simulink library "SLUGS_Library"  (Simulink 7.8)
settings: Solver=ode45  SolverMode=SingleTasking  StartTime=0.0  StopTime=10.0  RelTol=1e-3
values from neighbouring files (symbols this model uses):
  apSampleTime = 0.01    [mcuInit.m]
  derivativesConstant = 5    [mcuInit.m]
  latlong_WP = 1    [mcuInit.m]
  T = 0.01    [mcuInit.m]
  Xpoints = [0 0]    [mcuInit.m]
  Ypoints = [0 0]    [mcuInit.m]
  Zpoints = [0 0]    [mcuInit.m]
undefined symbols (not defined in the file or in its folder): bankCommandLimit, barAdjust, baroCutTemp, baroOffset, baroScale, barTGain1, barTGain2, barTMean1, barTMean2, baseHeight, baseTemp, daLimit, deLimit, DiscIntNeverNeededParam, drLimit, dtLimit, gaind, getGSLocation, getWP, GS_location, Init_onlyOnce, Init_Reset, IPStar, ISA_g, lapseRate, mass, maxAcc, MaxDwnPthStar, maxDynPressure, maxEta, Ndelay, param, pitAdjust, pitchCommandLimit, pitCutTemp, pitotOffset, pitotScale, pitTGain1, pitTGain2, pitTMean1, pitTMean2, polesd, pressureSensorCutoff, rollControlLimit, SampleT, setDiagnosticFloat, setDiagnosticShort, setLogFloat1, setLogFloat2, setNavLong, setNavNav, tanIntercept, Ts, u1, y1, yawDamperLimit, yo, zerosd
libraries: SLUGS_Library x90, simulink x37, dsPICdrivers x33, aerolibconvert2 x4, aerolibutil x1, aerolibobsolete x1
(part 2 of 7)

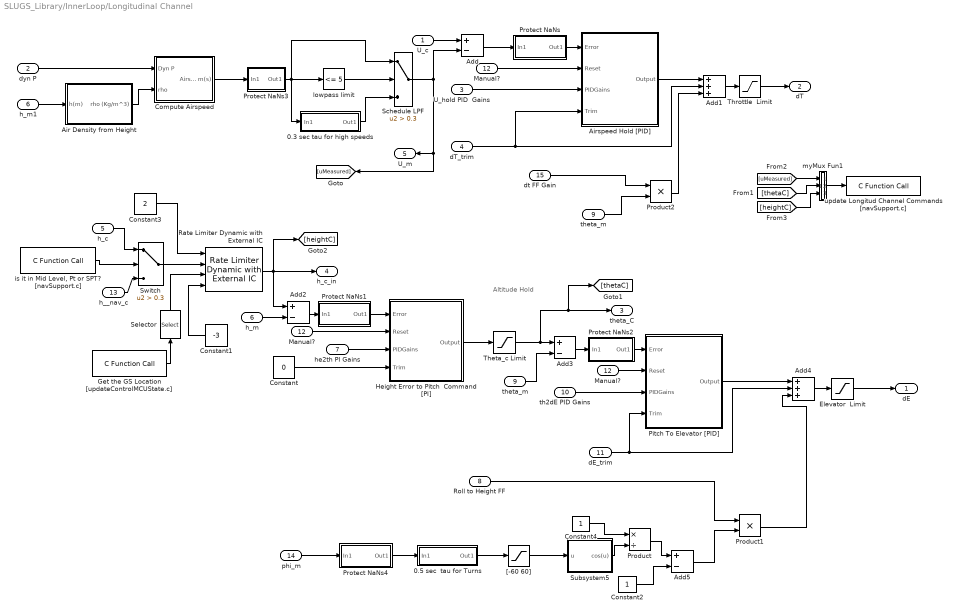
== system SLUGS_Library/InnerLoop/Longitudinal Channel ==
  note: Altitude Hold
  U_c : Inport
  dyn P : Inport  Port=2
  U_hold PID  Gains : Inport  Port=3
  dT_trim : Inport  Port=4
  h_c : Inport  Port=5
  h_m : Inport  Port=6
  he2th PI Gains : Inport  Port=7
  Roll to Height FF : Inport  Port=8
  theta_m : Inport  Port=9
  th2dE PID Gains : Inport  Port=10
  dE_trim : Inport  Port=11
  Manual? : Inport  Port=12
  h__nav_c : Inport  Port=13
  phi_m : Inport  Port=14
  dt FF Gain : Inport  Port=15
  " 0.3 sec tau for high speeds" : Subsystem  mask(Tustin1stOrderLowpassAutoInitialCondition){f=1, T=T}
      mask prompts: f "Lowpass Frequency"; T "Sample Time"
      mask help: Takes a 3db rolloff frequency (in Hz, NOT radians/s) and a sample time. Performs a symbolic Tustin conversion and implements in a discrete filter. The initial output of the filter is set by the first sample.
      mask Help: Enter the desired 3db rolloff frequency in Hz and the sample time. Initial conditions are sampled automatically.
      mask Display: fprintf('%.2f Hz lowpass',f)
  0.5 sec  tau for Turns : Subsystem  mask(Tustin1stOrderLowpassAutoInitialCondition){f=0.32, T=T}
      mask prompts: f "Lowpass Frequency"; T "Sample Time"
      mask help: Takes a 3db rolloff frequency (in Hz, NOT radians/s) and a sample time. Performs a symbolic Tustin conversion and implements in a discrete filter. The initial output of the filter is set by the first sample.
      mask Help: Enter the desired 3db rolloff frequency in Hz and the sample time. Initial conditions are sampled automatically.
      mask Display: fprintf('%.2f Hz lowpass',f)
  Add : Sum  Inputs=+-
  Add1 : Sum  Inputs=3  OutDataTypeStr=single
  Add2 : Sum  Inputs=+-  OutDataTypeStr=single
  Add3 : Sum  Inputs=+-  OutDataTypeStr=single
  Add4 : Sum  Inputs=3  OutDataTypeStr=single
  Add5 : Sum  Inputs=+-  OutDataTypeStr=single
  Air Density from Height : Subsystem  AncestorBlock=SLUGS_Library/Air Density from Height
  Airspeed Hold [PID] : Subsystem  AncestorBlock=SLUGS_Library/Control Blocks/PID Controller w//Anti-Windup  mask(PID){Tsample=apSampleTime, Ndelay=derivativesConstant, upperSaturationLimit=dtLimit, lowerSaturationLimit=0}
      mask prompts: Tsample "Sample Time"; Ndelay "Integer delays for de/dt"; upperSaturationLimit "Upper Saturation Limit"; lowerSaturationLimit "Lower Saturation Limit"
      mask help: PID controller block with anti-windup and saturation limits. Implemented as a discrete forwardl integration which stops integrating when the output is saturated. Derivative is implemented as a numerical derivative with N integer delays to smooth output.
      mask Display:
      | disp('PID')
      | port_label('input',1,'error')
      | port_label('input',3,'gains')
      | port_label('input',2,'reset')
      | port_label('input',4,'trim')
      | port_label('output',1,'output')
  Compute Airspeed : Subsystem  AncestorBlock=SLUGS_Library/Compute Airspeed
  Constant : Constant  Value=0
  Constant1 : Constant  Value=-3  OutDataTypeStr=single
  Constant2 : Constant  OutDataTypeStr=single
  Constant3 : Constant  Value=2  OutDataTypeStr=single
  Constant4 : Constant  OutDataTypeStr=single
  Elevator  Limit : Saturate  UpperLimit=deLimit  LowerLimit=-deLimit  SampleTime=apSampleTime
  Get the GS Location [updateControlMCUState.c] : dsPICdrivers/OTHERS/C Function Call  Tag=dsPIC_dsPIC_CFunctionCall  FctUpdate=Output Function  fctName='getGSLocation'  INPUT_SIZE=1  INPUT1=--  INPUT2=--  INPUT3=--  OUTPUT_SIZE=3  OUTPUT1=real32  SampleTime=0.01  InputType=[ ]  OutputType=[ 7 ]  FctDeclaration=extern void getGSLocation(real32_T* y1);  FctCall=getGSLocation(*%y1);  OrderingInOutPopup=None  FctStart=None  FctStart_Name=Init_onlyOnce  FctStart_Declaration=inline extern void Init_onlyOnce();  FctStart_Call=Init_onlyOnce();  FctInit=None  FctInit_Name=Init_Reset  FctInit_Declaration=inline extern void Init_Reset();  FctInit_Call=Init_Reset();  PinDigitalInput=[]  PinDigitalOutput=[]  AnalogueInput=[]
  Height Error to Pitch  Command [PI] : Subsystem  AncestorBlock=SLUGS_Library/Control Blocks/PI Controller w//Anti-Windup  mask(PID){Tsample=apSampleTime, Ndelay=derivativesConstant, upperSaturationLimit=pitchCommandLimit, lowerSaturationLimit=-pitchCommandLimit}
      mask prompts: Tsample "Sample Time"; Ndelay "Integer delays for de/dt"; upperSaturationLimit "Upper Saturation Limit"; lowerSaturationLimit "Lower Saturation Limit"
      mask help: PID controller block with anti-windup and saturation limits. Implemented as a discrete forwardl integration which stops integrating when the output is saturated. Derivative is implemented as a numerical derivative with N integer delays to smooth output.
      mask Display:
      | disp('PI')
      | port_label('input',1,'error')
      | port_label('input',3,'gains')
      | port_label('input',2,'reset')
      | port_label('input',4,'trim')
      | port_label('output',1,'output')
  "Manual? " : InportShadow  Port=12
  "Manual?  " : InportShadow  Port=12
  Pitch To Elevator [PID] : Subsystem  AncestorBlock=SLUGS_Library/Control Blocks/PID Controller w//Anti-Windup  mask(PID){Tsample=apSampleTime, Ndelay=derivativesConstant, upperSaturationLimit=deLimit, lowerSaturationLimit=-deLimit}
      mask prompts: Tsample "Sample Time"; Ndelay "Integer delays for de/dt"; upperSaturationLimit "Upper Saturation Limit"; lowerSaturationLimit "Lower Saturation Limit"
      mask help: PID controller block with anti-windup and saturation limits. Implemented as a discrete forwardl integration which stops integrating when the output is saturated. Derivative is implemented as a numerical derivative with N integer delays to smooth output.
      mask Display:
      | disp('PID')
      | port_label('input',1,'error')
      | port_label('input',3,'gains')
      | port_label('input',2,'reset')
      | port_label('input',4,'trim')
      | port_label('output',1,'output')
  Product : Product  Inputs=*/  RndMeth=Zero
  Product1 : Product  RndMeth=Zero
  Product2 : Product  RndMeth=Zero
  Protect NaNs : Subsystem
  Protect NaNs1 : Subsystem
  Protect NaNs2 : Subsystem
  Protect NaNs3 : Subsystem
  Protect NaNs4 : Subsystem
  Rate Limiter Dynamic with External IC : SLUGS_Library/Singnal Routing & Conditioning/Rate Limiter Dynamic with External IC  rlIC=0
  Schedule LPF : Switch  Criteria=u2 > Threshold  Threshold=0.3
  Selector : Selector  InputPortWidth=3  IndexOptions=Index vector (dialog)  Indices=[1 ]  OutputSizes=1
  Subsystem5 : Subsystem  AncestorBlock=SLUGS_Library/Subsystem5
  Switch : Switch  Criteria=u2 > Threshold  Threshold=0.3  OutDataTypeStr=Inherit: Inherit via back propagation  InputSameDT=on
  Theta_c Limit : Saturate  UpperLimit=pitchCommandLimit  LowerLimit=-pitchCommandLimit  SampleTime=apSampleTime
  Throttle  Limit : Saturate  UpperLimit=dtLimit  LowerLimit=0  SampleTime=apSampleTime
  "[-60 60]" : Saturate  UpperLimit=60  LowerLimit=-60  SampleTime=apSampleTime
  h_m1 : InportShadow  Port=6
  "is it in Mid Level, Pt or SPT? [navSupport.c]" : dsPICdrivers/OTHERS/C Function Call  Tag=dsPIC_dsPIC_CFunctionCall  FctUpdate=Output Function  fctName='isPassthrough'  INPUT_SIZE=1  INPUT1=--  INPUT2=--  INPUT3=--  OUTPUT_SIZE=1  OUTPUT1=uint8  SampleTime=0.01  InputType=[ ]  OutputType=[ 2 ]  FctDeclaration=extern uint8_T isPassthrough();  FctCall=%y1 = isPassthrough();  OrderingInOutPopup=None  FctStart=None  FctStart_Name=Init_onlyOnce  FctStart_Declaration=inline extern void Init_onlyOnce();  FctStart_Call=Init_onlyOnce();  FctInit=None  FctInit_Name=Init_Reset  FctInit_Declaration=inline extern void Init_Reset();  FctInit_Call=Init_Reset();  PinDigitalInput=[]  PinDigitalOutput=[]  AnalogueInput=[]
  lowpass limit : simulink/Logic and Bit Operations/Compare To Constant  relop=<=  const=5  OutDataTypeStr=uint8  ZeroCross=off
  myMux Fun1 : MATLAB Function  TreatAsAtomicUnit=on
  "theta_m " : InportShadow  Port=9
  update Longitud Channel Commands [navSupport.c] : dsPICdrivers/OTHERS/C Function Call  Tag=dsPIC_dsPIC_CFunctionCall  FctUpdate=Output Function  fctName='setNavLong'  INPUT_SIZE=3  INPUT1=real32  INPUT2=--  INPUT3=--  OUTPUT_SIZE=1  OUTPUT1=--  SampleTime=.01  InputType=[ 7 ]  OutputType=[ ]  FctDeclaration=extern void setNavLong(real32_T* u1);  FctCall=setNavLong(*%u1);  OrderingInOutPopup=None  FctStart=None  FctStart_Name=Init_onlyOnce  FctStart_Declaration=inline extern void Init_onlyOnce();  FctStart_Call=Init_onlyOnce();  FctInit=None  FctInit_Name=Init_Reset  FctInit_Declaration=inline extern void Init_Reset();  FctInit_Call=Init_Reset();  PinDigitalInput=[]  PinDigitalOutput=[]  AnalogueInput=[]
  dE : Outport
  dT : Outport  Port=2
  theta_C : Outport  Port=3
  h_c_in : Outport  Port=4
  U_m : Outport  Port=5
  wires:
  [heightC] -> myMux Fun1/3(u3)
  h_c/1 -> Switch/1
  h__nav_c/1 -> Switch/3
  Get the GS Location [updateControlMCUState.c]/1 -> Selector/1
  Protect NaNs4/1(Out1) -> 0.5 sec  tau for Turns/1(In1)
  Protect NaNs3/1(Out1) -> Schedule LPF/1, lowpass limit/1, " 0.3 sec tau for high speeds"/1(In1)
  Protect NaNs2/1(Out1) -> Pitch To Elevator [PID]/1(Error)
  Protect NaNs1/1(Out1) -> Height Error to Pitch  Command [PI]/1(Error)
  Protect NaNs/1(Out1) -> Airspeed Hold [PID]/1(Error)
  Constant/1 -> Height Error to Pitch  Command [PI]/4(Trim)
  U_hold PID  Gains/1 -> Airspeed Hold [PID]/3(PIDGains)
  dt FF Gain/1 -> Product2/1
  Product2/1 -> Add1/3
  "theta_m "/1 -> Product2/2
  Product1/1 -> Add4/3
  Roll to Height FF/1 -> Product1/1
  Add5/1 -> Product1/2
  "[-60 60]"/1 -> Subsystem5/1(u)
  0.5 sec  tau for Turns/1(Out1) -> "[-60 60]"/1
  Product/1 -> Add5/1
  Constant4/1 -> Product/1
  Subsystem5/1(cos(u)) -> Product/2
  Constant2/1 -> Add5/2
  phi_m/1 -> Protect NaNs4/1(In1)
  " 0.3 sec tau for high speeds"/1(Out1) -> Schedule LPF/3
  lowpass limit/1 -> Schedule LPF/2
  Compute Airspeed/1(Airspeed m(s)) -> Protect NaNs3/1(In1)
  Schedule LPF/1 -> [uMeasured], U_m/1, Add/2
  [thetaC] -> myMux Fun1/2(u2)
  [uMeasured] -> myMux Fun1/1(u1)
  myMux Fun1/1(y) -> update Longitud Channel Commands [navSupport.c]/1
  U_c/1 -> Add/1
  Add/1 -> Protect NaNs/1(In1)
  Airspeed Hold [PID]/1(Output) -> Add1/1
  dT_trim/1 -> Airspeed Hold [PID]/4(Trim), Add1/2
  Add1/1 -> Throttle  Limit/1
  Throttle  Limit/1 -> dT/1
  Add2/1 -> Protect NaNs1/1(In1)
  h_m/1 -> Add2/2
  theta_m/1 -> Add3/2
  Manual?/1 -> Airspeed Hold [PID]/2(Reset)
  "Manual? "/1 -> Height Error to Pitch  Command [PI]/2(Reset)
  "Manual?  "/1 -> Pitch To Elevator [PID]/2(Reset)
  Add4/1 -> Elevator  Limit/1
  Pitch To Elevator [PID]/1(Output) -> Add4/1
  dE_trim/1 -> Pitch To Elevator [PID]/4(Trim), Add4/2
  Elevator  Limit/1 -> dE/1
  Air Density from Height/1(rho (Kg/m^3)) -> Compute Airspeed/2(rho)
  dyn P/1 -> Compute Airspeed/1(Dyn P)
  h_m1/1 -> Air Density from Height/1(h(m))
  he2th PI Gains/1 -> Height Error to Pitch  Command [PI]/3(PIDGains)
  th2dE PID Gains/1 -> Pitch To Elevator [PID]/3(PIDGains)
  Add3/1 -> Protect NaNs2/1(In1)
  Theta_c Limit/1 -> [thetaC], theta_C/1, Add3/1
  "is it in Mid Level, Pt or SPT? [navSupport.c]"/1 -> Switch/2
  Rate Limiter Dynamic with External IC/1 -> [heightC], h_c_in/1, Add2/1
  Height Error to Pitch  Command [PI]/1(Output) -> Theta_c Limit/1
  Constant3/1 -> Rate Limiter Dynamic with External IC/1
  Switch/1 -> Rate Limiter Dynamic with External IC/2
  Selector/1 -> Rate Limiter Dynamic with External IC/3
  Constant1/1 -> Rate Limiter Dynamic with External IC/4

== system SLUGS_Library/InnerLoop/Navigation ==
  Puav : Inport  SampleTime=apSampleTime
  Max WP Idx : Inport  Port=2
  Vxyz : Inport  Port=3
  Start WP Idx : Inport  Port=4
  L1 Base (m) : Inport  Port=5
  R : Inport  Port=6
  WP Fly : Inport  Port=7
  Compute Lateral Error : SLUGS_Library/Navigation/Compute Lateral Error
  Compute WP Index : Subsystem  AncestorBlock=SLUGS_Library/Navigation/Compute WP Index
  Get Wps Compute Frenet : Subsystem
  "Park, Deyst & How Lat Accel Cmd" : SLUGS_Library/Navigation/Park, Deyst & How Lat Accel Cmd
  Selector : Selector  InputPortWidth=3  IndexOptions=Index vector (dialog)  Indices=[3]  OutputSizes=1
  To Workspace1 : ToWorkspace  VariableName=as_c  SampleTime=-1  SaveFormat=Array
  To Workspace2 : ToWorkspace  VariableName=N  SampleTime=-1  SaveFormat=Array
  To Workspace3 : ToWorkspace  VariableName=Phic  SampleTime=-1  SaveFormat=Array
  To Workspace4 : ToWorkspace  VariableName=T  SampleTime=-1  SaveFormat=Array
  UAV Weight : Constant  Value=mass  OutDataTypeStr=single
  UAV Pos1 : InportShadow  Port=1  SampleTime=apSampleTime
  as_c to phi_c : SLUGS_Library/Navigation/as_c to phi_c
  phi_c : Outport
  h_c : Outport  Port=2
  wires:
  Compute WP Index/2(WP0) -> Get Wps Compute Frenet/1(WP Idx 0)
  Compute WP Index/3(WP1) -> Get Wps Compute Frenet/2(WP Idx 1)
  Get Wps Compute Frenet/2(N) -> Compute Lateral Error/1, "Park, Deyst & How Lat Accel Cmd"/3, To Workspace2/1
  Get Wps Compute Frenet/1(T) -> To Workspace4/1, Compute WP Index/1(T1), "Park, Deyst & How Lat Accel Cmd"/2
  Puav/1 -> Compute WP Index/2(Puav)
  Max WP Idx/1 -> Compute WP Index/3(Max WP Index)
  Start WP Idx/1 -> Compute WP Index/4(StartingWP)
  "Park, Deyst & How Lat Accel Cmd"/1 -> To Workspace1/1, as_c to phi_c/1
  UAV Pos1/1 -> Compute Lateral Error/3
  as_c to phi_c/1 -> phi_c/1, To Workspace3/1
  UAV Weight/1 -> as_c to phi_c/2
  Compute Lateral Error/1 -> "Park, Deyst & How Lat Accel Cmd"/4
  Get Wps Compute Frenet/3(WP 1) -> Compute Lateral Error/2, Selector/1, Compute WP Index/5("WP1 ")
  Selector/1 -> h_c/1
  L1 Base (m)/1 -> "Park, Deyst & How Lat Accel Cmd"/5
  Compute WP Index/1(WP Change) -> Get Wps Compute Frenet/Enable
  R/1 -> Compute WP Index/6(R)
  Vxyz/1 -> "Park, Deyst & How Lat Accel Cmd"/1
  WP Fly/1 -> Compute WP Index/7(WP Fly)
  Compute WP Index/4(UAV IC) -> Get Wps Compute Frenet/3(UAV IC)

== system SLUGS_Library/Navigation/Bank to Psi Dot ==
  phi_c : Inport
  U_m : Inport  Port=2
  Constant1 : Constant  Value=9.80665  OutDataTypeStr=single
  Divide : Product  Inputs=/*  OutDataTypeStr=single
  Divide1 : Product  OutDataTypeStr=single
  Subsystem8 : SLUGS_Library/Subsystem8
  negprotect : MATLAB Function  TreatAsAtomicUnit=on
  psi_dot_c : Outport
  wires:
  U_m/1 -> negprotect/1(val)
  Constant1/1 -> Divide/2
  Divide1/1 -> psi_dot_c/1
  Subsystem8/1 -> Divide1/1
  phi_c/1 -> Subsystem8/1
  Divide/1 -> Divide1/2
  negprotect/1(zpVal) -> Divide/1

== system SLUGS_Library/Navigation/Compute Lateral Error ==
  N : Inport
  WP1 : Inport  Port=2
  UAV pos : Inport  Port=3
  Add : Sum  Inputs=+-
  Subsystem3 : SLUGS_Library/Subsystem3
  Pe_lat : Outport
  wires:
  WP1/1 -> Add/1
  UAV pos/1 -> Add/2
  N/1 -> Subsystem3/1
  Add/1 -> Subsystem3/2
  Subsystem3/1 -> Pe_lat/1

== system SLUGS_Library/Navigation/Compute Distance ==
  Pos 1 : Inport
  Pos 2 : Inport  Port=2
  Add : Sum  Inputs=+-
  Norm : SLUGS_Library/Navigation/Norm
  Dist : Outport
  wires:
  Pos 1/1 -> Add/1
  Pos 2/1 -> Add/2
  Add/1 -> Norm/1
  Norm/1 -> Dist/1

== system SLUGS_Library/Navigation/Compute Frenet ==
  Pos 1 : Inport
  Pos 2 : Inport  Port=2
  Add : Sum  Inputs=-+
  Normalize Vector : SLUGS_Library/Navigation/Normalize Vector
  "Normalize Vector " : SLUGS_Library/Navigation/Normalize Vector
  Select N  Terms : MATLAB Function  TreatAsAtomicUnit=on
  T : Outport
  N : Outport  Port=2
  wires:
  Pos 1/1 -> Add/1
  Pos 2/1 -> Add/2
  Add/1 -> Normalize Vector/1
  Normalize Vector/1 -> T/1, Select N  Terms/1(T)
  Select N  Terms/1(N) -> "Normalize Vector "/1
  "Normalize Vector "/1 -> N/1

== system SLUGS_Library/Navigation/Compute WP Index ==
  T1 : Inport
  Puav : Inport  Port=2
  Max WP Index : Inport  Port=3
  StartingWP : Inport  Port=4
  "WP1 " : Inport  Port=5
  R : Inport  Port=6
  WP Fly : Inport  Port=7
  Add : Sum  Inputs=2
  Compute Distance : SLUGS_Library/Navigation/Compute Distance
  Compute Modified L1 : Subsystem
  Data Type Conversion : DataTypeConversion  OutDataTypeStr=double  SampleTime=apSampleTime
  Embedded MATLAB Function : MATLAB Function  TreatAsAtomicUnit=on
  Enabled Subsystem : Subsystem  TreatAsAtomicUnit=on
  Hit  Crossing : HitCross  HitCrossingOffset=0.9  HitCrossingDirection=rising  SampleTime=apSampleTime
  IC : InitialCondition
  IC1 : InitialCondition  Value=0
  Integer Delay : Delay  DelayLength=1  InputProcessing=Inherited
  Integer Delay2 : Delay  DelayLength=1  InitialCondition=0  InputProcessing=Inherited
  Integer Delay3 : Delay  DelayLength=1  InitialCondition=150  InputProcessing=Inherited
  Logical Operator : Logic  Operator=OR  AllPortsSameDT=off  OutDataTypeStr=boolean
  "Puav " : InportShadow  Port=2
  Subsystem : Subsystem
  Switch Distance Less than? : RelationalOperator  OutDataTypeStr=boolean  SampleTime=apSampleTime
  WP1 1 : InportShadow  Port=5
  WP Change : Outport
  WP0 : Outport  Port=2
  WP1 : Outport  Port=3
  UAV IC : Outport  Port=4
  wires:
  Integer Delay/1 -> Compute Distance/2  "next WP"
  Puav/1 -> Compute Distance/1
  Embedded MATLAB Function/2(wp1) -> WP1/1
  Embedded MATLAB Function/1(wp0) -> WP0/1
  StartingWP/1 -> Embedded MATLAB Function/1(wpStart)
  Switch Distance Less than?/1 -> Data Type Conversion/1
  Max WP Index/1 -> Embedded MATLAB Function/2(wpCount)
  Compute Distance/1 -> Switch Distance Less than?/2
  "WP1 "/1 -> Integer Delay/1
  Hit  Crossing/1 -> Embedded MATLAB Function/3(swIncrement), IC/1
  Data Type Conversion/1 -> Hit  Crossing/1
  Embedded MATLAB Function/3(wp2) -> Compute Modified L1/3(WP2)
  WP1 1/1 -> Compute Modified L1/1(WP1)
  T1/1 -> Compute Modified L1/2(T1)
  Integer Delay2/1 -> Add/1
  Add/1 -> Compute Modified L1/Enable, Logical Operator/1
  IC/1 -> Add/2, Integer Delay2/1
  Compute Modified L1/1(P) -> Integer Delay3/1
  Integer Delay3/1 -> Switch Distance Less than?/1
  R/1 -> Compute Modified L1/4(R)
  WP Fly/1 -> IC1/1
  Subsystem/1(Just Enab) -> Enabled Subsystem/Enable, [WpEnabl]
  "Puav "/1 -> Enabled Subsystem/1(In1)
  Enabled Subsystem/1(Out1) -> UAV IC/1
  IC1/1 -> Subsystem/1(WP Fly)
  [WpEnabl] -> Embedded MATLAB Function/4(wpEnabl)
  Logical Operator/1 -> WP Change/1
  [WpEnabl] -> Logical Operator/2

== system SLUGS_Library/Navigation/Geod2LTP ==
  GS Lat,Lon : Inport
  GS ECEF : Inport  Port=2
  "Lat, deg(GPS)" : Inport  Port=3
  "Lon, deg(GPS)" : Inport  Port=4
  Hight,m(GPS) : Inport  Port=5
  ECEF2LTP (UEN) : Subsystem
      mask Display: plot(0,0,100,100,[45,40,35,40,40],[85,95,85,95,40],[85,95,85,95,40],[35,40,45,40,40],[60,40,10,20,10,14],[70,40,10,13,10,20],[56,45],[70,70],[60,60],[50,60],[60,60],[30,40],[50,60],[20,20],[30,40],[20,20],[45,55],[35,25],[75,65],[35,25])
  Geod2ECEF1 : Subsystem  mask{Re=6378137, Rp=6356752.3142}
      mask prompts: Re "Enter equatorial radius, m"; Rp "Enter polar radius,m"
  Mux : Mux  Inputs=3
  Reshape : Reshape  OutputDimensionality=Column vector (2-D)
  Reshape1 : Reshape
  Sum1 : Sum  Inputs=|+-  OutDataTypeStr=single  SaturateOnIntegerOverflow=on
  UEN 2 NEU : Gain  Gain=[0 0 1;0 1 0;1 0 0]  Multiplication=Matrix(K*u)  OutDataTypeStr=float('single')  SaturateOnIntegerOverflow=on  ParamDataTypeStr=Inherit: Same as input
  "NEU, m" : Outport
  wires:
  Reshape1/1 -> "NEU, m"/1
  Reshape/1 -> UEN 2 NEU/1
  Sum1/1 -> ECEF2LTP (UEN)/1(ECEF coordinates)
  Mux/1 -> Sum1/1  "r_mov"
  Hight,m(GPS)/1 -> Geod2ECEF1/1("height, m")
  ECEF2LTP (UEN)/1(Out) -> Reshape/1  "Moving Side"
  GS ECEF/1 -> Sum1/2
  GS Lat,Lon/1 -> ECEF2LTP (UEN)/2("Long, Lat")
  "Lon, deg(GPS)"/1 -> Geod2ECEF1/3(lon,deg)
  "Lat, deg(GPS)"/1 -> Geod2ECEF1/2("lat, deg")
  Geod2ECEF1/2("Ye, m ") -> Mux/2
  Geod2ECEF1/1("Xe, m ") -> Mux/1
  Geod2ECEF1/3("Ze, m ") -> Mux/3
  UEN 2 NEU/1 -> Reshape1/1

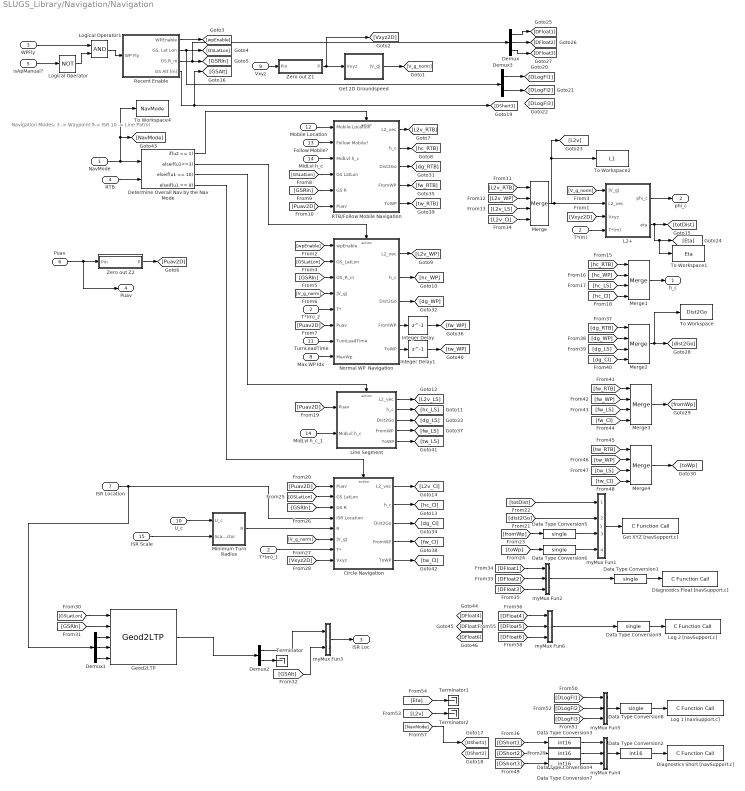
== system SLUGS_Library/Navigation/Navigation ==
  note: Navigation Modes:
      | 3 -> Waypoint
      | 9-> ISR
      | 10 -> Line Patrol
  NavMode : Inport
  T*(m) : Inport  Port=2
  WPFly : Inport  Port=3
  RTB : Inport  Port=4
  isApManual? : Inport  Port=5
  Puav : Inport  Port=6  SampleTime=apSampleTime
  ISR Location : Inport  Port=7
  Max WP Idx : Inport  Port=8
  Vxyz : Inport  Port=9  SampleTime=apSampleTime
  U_c : Inport  Port=10
  TurnLeadTime : Inport  Port=11
  Mobile Location : Inport  Port=12
  Follow Mobile? : Inport  Port=13
  MidLvl h_c : Inport  Port=14
  ISR Scale : Inport  Port=15
  Circle Navigation : Subsystem  TreatAsAtomicUnit=on
  Data Type Conversion{1,5..6,8..9} (5 alike) : DataTypeConversion  OutDataTypeStr=single
  Data Type Conversion{2..4,7} (4 alike) : DataTypeConversion  OutDataTypeStr=int16
  Demux : Demux  Outputs=3
  Demux1 : Demux  Outputs=3
  Demux2 : Demux  Outputs=[2 1]
  Demux3 : Demux  Outputs=2
  Determine Overall Nav by the Nav Mode : If  NumInputs=2  IfExpression=u2 == 1  ElseIfExpressions=u1==3, u1 == 10, u1 == 9  ShowElse=off
  Diagnostics Float [navSupport.c] : dsPICdrivers/OTHERS/C Function Call  Tag=dsPIC_dsPIC_CFunctionCall  FctUpdate=Output Function  fctName='setDiagnosticFloat'  INPUT_SIZE=3  INPUT1=real32  INPUT2=--  INPUT3=--  OUTPUT_SIZE=1  OUTPUT1=--  SampleTime=.01  InputType=[ 7 ]  OutputType=[ ]  FctDeclaration=extern void setDiagnosticFloat(real32_T* u1);  FctCall=setDiagnosticFloat(*%u1);  OrderingInOutPopup=None  FctStart=None  FctStart_Name=Init_onlyOnce  FctStart_Declaration=inline extern void Init_onlyOnce();  FctStart_Call=Init_onlyOnce();  FctInit=None  FctInit_Name=Init_Reset  FctInit_Declaration=inline extern void Init_Reset();  FctInit_Call=Init_Reset();  PinDigitalInput=[]  PinDigitalOutput=[]  AnalogueInput=[]
  Diagnostics Short [navSupport.c] : dsPICdrivers/OTHERS/C Function Call  Tag=dsPIC_dsPIC_CFunctionCall  FctUpdate=Output Function  fctName='setDiagnosticShort'  INPUT_SIZE=3  INPUT1=int16  INPUT2=--  INPUT3=--  OUTPUT_SIZE=1  OUTPUT1=--  SampleTime=.01  InputType=[ 3 ]  OutputType=[ ]  FctDeclaration=extern void setDiagnosticShort(int16_T* u1);  FctCall=setDiagnosticShort(*%u1);  OrderingInOutPopup=None  FctStart=None  FctStart_Name=Init_onlyOnce  FctStart_Declaration=inline extern void Init_onlyOnce();  FctStart_Call=Init_onlyOnce();  FctInit=None  FctInit_Name=Init_Reset  FctInit_Declaration=inline extern void Init_Reset();  FctInit_Call=Init_Reset();  PinDigitalInput=[]  PinDigitalOutput=[]  AnalogueInput=[]
  Geod2LTP : SLUGS_Library/Navigation/Geod2LTP
  Get 2D Groundspeed : Subsystem
  Get XYZ [navSupport.c] : dsPICdrivers/OTHERS/C Function Call  Tag=dsPIC_dsPIC_CFunctionCall  FctUpdate=Output Function  fctName='setNavNav'  INPUT_SIZE=4  INPUT1=real32  INPUT2=--  INPUT3=--  OUTPUT_SIZE=1  OUTPUT1=--  SampleTime=.01  InputType=[ 7 ]  OutputType=[ ]  FctDeclaration=extern void setNavNav(real32_T* u1);  FctCall=setNavNav(*%u1);  OrderingInOutPopup=None  FctStart=None  FctStart_Name=Init_onlyOnce  FctStart_Declaration=inline extern void Init_onlyOnce();  FctStart_Call=Init_onlyOnce();  FctInit=None  FctInit_Name=Init_Reset  FctInit_Declaration=inline extern void Init_Reset();  FctInit_Call=Init_Reset();  PinDigitalInput=[]  PinDigitalOutput=[]  AnalogueInput=[]
  Integer Delay : Delay  DelayLength=1  InputProcessing=Inherited
  Integer Delay1 : Delay  DelayLength=1  InputProcessing=Inherited
  L2+ : Subsystem
  Line Segment : Subsystem  TreatAsAtomicUnit=on
  Log 1 [navSupport.c] : dsPICdrivers/OTHERS/C Function Call  Tag=dsPIC_dsPIC_CFunctionCall  FctUpdate=Output Function  fctName='setLogFloat1'  INPUT_SIZE=3  INPUT1=real32  INPUT2=--  INPUT3=--  OUTPUT_SIZE=1  OUTPUT1=--  SampleTime=.01  InputType=[ 7 ]  OutputType=[ ]  FctDeclaration=extern void setLogFloat1(real32_T* u1);  FctCall=setLogFloat1(*%u1);  OrderingInOutPopup=None  FctStart=None  FctStart_Name=Init_onlyOnce  FctStart_Declaration=inline extern void Init_onlyOnce();  FctStart_Call=Init_onlyOnce();  FctInit=None  FctInit_Name=Init_Reset  FctInit_Declaration=inline extern void Init_Reset();  FctInit_Call=Init_Reset();  PinDigitalInput=[]  PinDigitalOutput=[]  AnalogueInput=[]
  Log 2 [navSupport.c] : dsPICdrivers/OTHERS/C Function Call  Tag=dsPIC_dsPIC_CFunctionCall  FctUpdate=Output Function  fctName='setLogFloat2'  INPUT_SIZE=3  INPUT1=real32  INPUT2=--  INPUT3=--  OUTPUT_SIZE=1  OUTPUT1=--  SampleTime=.01  InputType=[ 7 ]  OutputType=[ ]  FctDeclaration=extern void setLogFloat2(real32_T* u1);  FctCall=setLogFloat2(*%u1);  OrderingInOutPopup=None  FctStart=None  FctStart_Name=Init_onlyOnce  FctStart_Declaration=inline extern void Init_onlyOnce();  FctStart_Call=Init_onlyOnce();  FctInit=None  FctInit_Name=Init_Reset  FctInit_Declaration=inline extern void Init_Reset();  FctInit_Call=Init_Reset();  PinDigitalInput=[]  PinDigitalOutput=[]  AnalogueInput=[]
  Logical Operator : Logic  Operator=NOT  AllPortsSameDT=off  OutDataTypeStr=boolean
  Logical Operator1 : Logic  AllPortsSameDT=off  OutDataTypeStr=boolean
  Merge{,1..4} (5 alike) : Merge  Inputs=4
  MidLvl h_c_1 : InportShadow  Port=14
  Minimum Turn Radius : Subsystem
  Normal WP  Navigation : Subsystem  TreatAsAtomicUnit=on
  RTB/Follow Mobile Navigation : Subsystem
  Recent Enable : Subsystem
  T*(m)_1 : InportShadow  Port=2
  T*(m)_2 : InportShadow  Port=2
  Terminator : Terminator
  Terminator1 : Terminator
  Terminator2 : Terminator
  To Workspace : ToWorkspace  VariableName=Dist2Go  SampleTime=-1  SaveFormat=Array
  To Workspace1 : ToWorkspace  VariableName=Eta  SampleTime=-1  SaveFormat=Array
  To Workspace2 : ToWorkspace  VariableName=L1  SampleTime=-1  SaveFormat=Array
  To Workspace4 : ToWorkspace  VariableName=NavMode  SampleTime=-1  SaveFormat=Array
  Zero out Z1 : MATLAB Function  TreatAsAtomicUnit=on
  Zero out Z2 : MATLAB Function  TreatAsAtomicUnit=on
  myMux Fun1 : MATLAB Function  TreatAsAtomicUnit=on
  myMux Fun2 : MATLAB Function  TreatAsAtomicUnit=on
  myMux Fun3 : MATLAB Function  TreatAsAtomicUnit=on
  myMux Fun4 : MATLAB Function  TreatAsAtomicUnit=on
  myMux Fun5 : MATLAB Function  TreatAsAtomicUnit=on
  myMux Fun6 : MATLAB Function  TreatAsAtomicUnit=on
  h_c : Outport
  phi_c : Outport  Port=2
  ISR Loc : Outport  Port=3
  "Puav " : Outport  Port=4
  wires:
  Data Type Conversion9/1 -> Log 2 [navSupport.c]/1
  myMux Fun6/1(y) -> Data Type Conversion9/1
  [DFloat5] -> myMux Fun6/2(u2)
  [DFloat4] -> myMux Fun6/1(u1)
  [DFloat6] -> myMux Fun6/3(u3)
  Recent Enable/4(GS Alt (m)) -> [GSAlt], [DShort3]
  Demux/3 -> [DFloat3]
  [NavMode] -> [DShort1]
  Demux3/2 -> [DLogFl2]
  Demux3/1 -> [DLogFl1]
  Demux/2 -> [DFloat2]
  Demux/1 -> [DFloat1]
  [L2v] -> Terminator2/1
  [Eta] -> Terminator1/1
  myMux Fun2/1(y) -> Data Type Conversion1/1
  WPFly/1 -> Logical Operator1/1
  Logical Operator/1 -> Logical Operator1/2
  Logical Operator1/1 -> Recent Enable/1(WP Fly)
  isApManual?/1 -> Logical Operator/1
  MidLvl h_c_1/1 -> Line Segment/2(MidLvl h_c)
  [Puav2D] -> Line Segment/1(Puav)
  [hc_CI] -> Merge1/4
  [hc_LS] -> Merge1/3
  [hc_WP] -> Merge1/2
  [hc_RTB] -> Merge1/1
  [L2v_CI] -> Merge/4
  [L2v_LS] -> Merge/3
  [L2v_WP] -> Merge/2
  [L2v_RTB] -> Merge/1
  Line Segment/2(h_c) -> [hc_LS]
  Line Segment/1(L2_vec) -> [L2v_LS]
  Normal WP  Navigation/2(h_c) -> [hc_WP]
  Normal WP  Navigation/1(L2_vec) -> [L2v_WP]
  RTB/Follow Mobile Navigation/2(h_c) -> [hc_RTB]
  RTB/Follow Mobile Navigation/1(L2_vec) -> [L2v_RTB]
  Merge1/1 -> h_c/1
  [Puav2D] -> RTB/Follow Mobile Navigation/6(Puav)
  Zero out Z2/1(P) -> [Puav2D]
  [GSRIn] -> RTB/Follow Mobile Navigation/5(GS R)
  [GSLatLon] -> RTB/Follow Mobile Navigation/4(GS LatLon)
  Max WP Idx/1 -> Normal WP  Navigation/8(MaxWp)
  TurnLeadTime/1 -> Normal WP  Navigation/7(TurnLeadTime)
  [Puav2D] -> Normal WP  Navigation/6(Puav)
  T*(m)_2/1 -> Normal WP  Navigation/5(T*)
  [V_g_norm] -> Normal WP  Navigation/4(|V_g|)
  [wpEnable] -> Normal WP  Navigation/1(wpEnable)
  [GSLatLon] -> Normal WP  Navigation/2(GS_LatLon)
  [GSRIn] -> Normal WP  Navigation/3(GS_R_in)
  Puav/1 -> Zero out Z2/1(Pin), "Puav "/1
  Zero out Z1/1(P) -> [Vxyz2D], Get 2D Groundspeed/1(Vxyz)
  Determine Overall Nav by the Nav Mode/1 -> RTB/Follow Mobile Navigation/Action
  Mobile Location/1 -> RTB/Follow Mobile Navigation/1(Mobile Location)
  MidLvl h_c/1 -> RTB/Follow Mobile Navigation/3(MidLvl h_c)
  Follow Mobile?/1 -> RTB/Follow Mobile Navigation/2(Follow Mobile?)
  RTB/1 -> Determine Overall Nav by the Nav Mode/2
  Determine Overall Nav by the Nav Mode/4 -> Circle Navigation/Action
  Determine Overall Nav by the Nav Mode/2 -> Normal WP  Navigation/Action
  Recent Enable/3(GS R_in) -> Demux/1, [GSRIn]
  Recent Enable/2("GS, Lat Lon") -> Demux3/1, [GSLatLon]
  Recent Enable/1(WPEnable) -> [wpEnable]
  Merge/1 -> To Workspace2/1, [L2v], L2+/2(L2_vec)
  NavMode/1 -> To Workspace4/1, [NavMode], Determine Overall Nav by the Nav Mode/1
  T*(m)/1 -> L2+/4(T*(m))
  L2+/1(phi_c) -> phi_c/1
  [V_g_norm] -> L2+/1(|V_g|)
  [Vxyz2D] -> L2+/3(Vxyz)
  Get 2D Groundspeed/1(|V_g|) -> [V_g_norm]
  Vxyz/1 -> Zero out Z1/1(Pin)
  myMux Fun1/1(y) -> Get XYZ [navSupport.c]/1
  [totDist] -> myMux Fun1/1(u1)
  [dist2Go] -> myMux Fun1/2(u2)
  [fromWp] -> Data Type Conversion5/1
  [toWp] -> Data Type Conversion6/1
  Data Type Conversion5/1 -> myMux Fun1/3(u3)
  Data Type Conversion6/1 -> myMux Fun1/4(u4)
  L2+/2(eta) -> To Workspace1/1, [Eta], [totDist]
  [dg_CI] -> Merge2/4
  [dg_LS] -> Merge2/3
  [dg_WP] -> Merge2/2
  [dg_RTB] -> Merge2/1
  [fw_CI] -> Merge3/4
  [fw_LS] -> Merge3/3
  [fw_WP] -> Merge3/2
  [fw_RTB] -> Merge3/1
  [tw_CI] -> Merge4/4
  [tw_LS] -> Merge4/3
  [tw_WP] -> Merge4/2
  [tw_RTB] -> Merge4/1
  Merge2/1 -> To Workspace/1, [dist2Go]
  Merge4/1 -> [toWp]
  Merge3/1 -> [fromWp]
  RTB/Follow Mobile Navigation/3(Dist2Go) -> [dg_RTB]
  Normal WP  Navigation/3(Dist2Go) -> [dg_WP]
  Line Segment/3(Dist2Go) -> [dg_LS]
  RTB/Follow Mobile Navigation/4(FromWP) -> [fw_RTB]
  Normal WP  Navigation/4(FromWP) -> Integer Delay/1
  Line Segment/4(FromWP) -> [fw_LS]
  RTB/Follow Mobile Navigation/5(ToWP) -> [tw_RTB]
  Normal WP  Navigation/5(ToWP) -> Integer Delay1/1
  Line Segment/5(ToWP) -> [tw_LS]
  Integer Delay/1 -> [fw_WP]
  Integer Delay1/1 -> [tw_WP]
  [Puav2D] -> Circle Navigation/1(Puav)
  Circle Navigation/2(h_c) -> [hc_CI]
  Circle Navigation/1(L2_vec) -> [L2v_CI]
  Circle Navigation/3(Dist2Go) -> [dg_CI]
  Circle Navigation/4(FromWP) -> [fw_CI]
  Circle Navigation/5(ToWP) -> [tw_CI]
  [GSLatLon] -> Circle Navigation/2(GS LatLon)
  [GSRIn] -> Circle Navigation/3(GS R)
  Minimum Turn Radius/1(R) -> Circle Navigation/5(R)
  [V_g_norm] -> Circle Navigation/6(|V_g|)
  T*(m)_1/1 -> Circle Navigation/7(T*)
  [Vxyz2D] -> Circle Navigation/8(Vxyz)
  ISR Location/1 -> Circle Navigation/4(ISR Location), Demux1/1
  U_c/1 -> Minimum Turn Radius/1(U_c)
  Determine Overall Nav by the Nav Mode/3 -> Line Segment/Action
  ISR Scale/1 -> Minimum Turn Radius/2(Scale Factor)
  [DFloat2] -> myMux Fun2/2(u2)
  [DFloat1] -> myMux Fun2/1(u1)
  [DFloat3] -> myMux Fun2/3(u3)
  Data Type Conversion1/1 -> Diagnostics Float [navSupport.c]/1
  Demux1/1 -> Geod2LTP/3
  Demux1/2 -> Geod2LTP/4
  Demux1/3 -> Geod2LTP/5
  [GSLatLon] -> Geod2LTP/1
  [GSRIn] -> Geod2LTP/2
  myMux Fun3/1(y) -> ISR Loc/1
  Demux2/1 -> myMux Fun3/1(u1)
  Demux2/2 -> Terminator/1
  Geod2LTP/1 -> Demux2/1
  [GSAlt] -> myMux Fun3/2(u2)
  Data Type Conversion2/1 -> Diagnostics Short [navSupport.c]/1
  myMux Fun4/1(y) -> Data Type Conversion2/1
  [DShort2] -> Data Type Conversion4/1
  [DShort1] -> Data Type Conversion3/1
  [DShort3] -> Data Type Conversion7/1
  Data Type Conversion3/1 -> myMux Fun4/1(u1)
  Data Type Conversion4/1 -> myMux Fun4/2(u2)
  Data Type Conversion7/1 -> myMux Fun4/3(u3)
  myMux Fun5/1(y) -> Data Type Conversion8/1
  [DLogFl3] -> myMux Fun5/3(u3)
  [DLogFl2] -> myMux Fun5/2(u2)
  [DLogFl1] -> myMux Fun5/1(u1)
  Data Type Conversion8/1 -> Log 1 [navSupport.c]/1

== system SLUGS_Library/Navigation/Norm ==
  Vector : Inport
  Subsystem1 : SLUGS_Library/Subsystem1
  Subsystem3 : SLUGS_Library/Subsystem3
  Norm : Outport
  wires:
  Subsystem3/1 -> Subsystem1/1
  Vector/1 -> Subsystem3/2, Subsystem3/1
  Subsystem1/1 -> Norm/1

== system SLUGS_Library/Navigation/Normalize Vector ==
  Vector : Inport
  Divide : Product  Inputs=*/
  Vector Norm : SLUGS_Library/Vector Norm
  Zero Bound : Saturate  UpperLimit=inf  LowerLimit=0.001
  Normalized : Outport
  wires:
  Divide/1 -> Normalized/1
  Zero Bound/1 -> Divide/2
  Vector Norm/1 -> Zero Bound/1
  Vector/1 -> Divide/1, Vector Norm/1

== system SLUGS_Library/Navigation/Park, Deyst & How Lat Accel Cmd ==
  Vxyz : Inport
  T : Inport  Port=2
  N : Inport  Port=3
  Pe_lat : Inport  Port=4
  L1 : Inport  Port=5
  Compute Eta : Subsystem
  Compute L1 Vector LINE MODE : Subsystem
  "L1 " : InportShadow  Port=5
  Park's Lateral Accel Command : Subsystem
  a_s_c : Outport
  wires:
  Park's Lateral Accel Command/1(a_s_c) -> a_s_c/1
  Compute L1 Vector LINE MODE/1(L1_vec) -> Compute Eta/2(L1_vec)
  Compute Eta/1(Eta) -> Park's Lateral Accel Command/3(eta)
  Vxyz/1 -> Compute Eta/1(Vxyz), Park's Lateral Accel Command/1(Vxyz)
  "L1 "/1 -> Park's Lateral Accel Command/2(L1)
  Pe_lat/1 -> Compute L1 Vector LINE MODE/1(Pe_lat)
  L1/1 -> Compute L1 Vector LINE MODE/2(L1)
  T/1 -> Compute L1 Vector LINE MODE/3(T)
  N/1 -> Compute L1 Vector LINE MODE/4(N)

== system SLUGS_Library/Navigation/as_c to phi_c ==
  as_c : Inport
  W : Inport  Port=2
  Divide : Product  Inputs=*/
  Subsystem2 : SLUGS_Library/Subsystem2
  phi_c : Outport
  wires:
  Divide/1 -> Subsystem2/1
  as_c/1 -> Divide/1
  Subsystem2/1 -> phi_c/1
  W/1 -> Divide/2

== system SLUGS_Library/Navigation/get WP Coord from Index ==
  WP Idx : Inport
  GS LLA : Inport  Port=2
  GS R_in : Inport  Port=3
  Demux1 : Demux  Outputs=3
  Environment Controller1 : simulink/Signal Routing/Environment Controller
  Geod2LTP2 : SLUGS_Library/Navigation/Geod2LTP
  Get WP from idx SIM : Subsystem
  Get Waypoint Coordinates [navSupport.c] : dsPICdrivers/OTHERS/C Function Call  Tag=dsPIC_dsPIC_CFunctionCall  FctUpdate=Output Function  fctName='getWP'  INPUT_SIZE=1  INPUT1=uint8  INPUT2=--  INPUT3=--  OUTPUT_SIZE=3  OUTPUT1=real32  SampleTime=-1  InputType=[ 2 ]  OutputType=[ 7 ]  FctDeclaration=extern void getWP(uint8_T u1,real32_T* y1);  FctCall=getWP(%u1, *%y1);  OrderingInOutPopup=None  FctStart=None  FctStart_Name=Init_onlyOnce  FctStart_Declaration=inline extern void Init_onlyOnce();  FctStart_Call=Init_onlyOnce();  FctInit=None  FctInit_Name=Init_Reset  FctInit_Declaration=inline extern void Init_Reset();  FctInit_Call=Init_Reset();  PinDigitalInput=[]  PinDigitalOutput=[]  AnalogueInput=[]
  WP Coord : Outport
  wires:
  WP Idx/1 -> Get Waypoint Coordinates [navSupport.c]/1, Get WP from idx SIM/3(idx)
  GS LLA/1 -> Geod2LTP2/1, Get WP from idx SIM/1(GS LLA)
  GS R_in/1 -> Geod2LTP2/2, Get WP from idx SIM/2(GS ECEF)
  Environment Controller1/1 -> WP Coord/1
  Get WP from idx SIM/1(Out1) -> Environment Controller1/1
  Demux1/1 -> Geod2LTP2/3
  Demux1/2 -> Geod2LTP2/4
  Demux1/3 -> Geod2LTP2/5
  Get Waypoint Coordinates [navSupport.c]/1 -> Demux1/1
  Geod2LTP2/1 -> Environment Controller1/2

== system SLUGS_Library/Navigation/psi_dot to Bank ==
  psi_dot_c : Inport
  U_m : Inport  Port=2
  Constant1 : Constant  Value=9.80665  OutDataTypeStr=single
  Divide : Product  Inputs=**/
  dsPIC_atan : SLUGS_Library/dsPIC_atan
  phi_c : Outport
  wires:
  psi_dot_c/1 -> Divide/1
  U_m/1 -> Divide/2
  Constant1/1 -> Divide/3
  dsPIC_atan/1 -> phi_c/1
  Divide/1 -> dsPIC_atan/1

== system SLUGS_Library/Sensor Blocks/Baro Alt ==
  Baro raw : Inport
  Temperature : Inport  Port=2
  Baro Altimeter : Subsystem
  Barometer Unit Conversion : Subsystem  mask{bias=baroOffset, gains=baroScale}
      mask prompts: bias "Initial Bias"; gains "Initial Gains"
      mask help: Convert Analog readings to units
  Data Type Conversion2 : DataTypeConversion  OutDataTypeStr=single
  Data Type Conversion3 : DataTypeConversion  OutDataTypeStr=double
  Temp Compensate Baro : Subsystem
  "Tustin Lowpass, Auto Initial Condition" : Subsystem  mask(Tustin1stOrderLowpassAutoInitialCondition){f=pressureSensorCutoff, T=apSampleTime}
      mask prompts: f "Lowpass Frequency"; T "Sample Time"
      mask help: Takes a 3db rolloff frequency (in Hz, NOT radians/s) and a sample time. Performs a symbolic Tustin conversion and implements in a discrete filter. The initial output of the filter is set by the first sample.
      mask Help: Enter the desired 3db rolloff frequency in Hz and the sample time. Initial conditions are sampled automatically.
      mask Display: fprintf('%.2f Hz lowpass',f)
  Baro Alt (m) : Outport
  Static (Pa) : Outport  Port=2
  wires:
  Data Type Conversion3/1 -> "Tustin Lowpass, Auto Initial Condition"/1(In1)
  Barometer Unit Conversion/1(Comp) -> Baro Altimeter/1(Static (Pa)), Static (Pa)/1
  "Tustin Lowpass, Auto Initial Condition"/1(Out1) -> Data Type Conversion2/1
  Data Type Conversion2/1 -> Barometer Unit Conversion/1(Raw)
  Temp Compensate Baro/1(Baro_c) -> Data Type Conversion3/1
  Baro raw/1 -> Temp Compensate Baro/2(Baro)
  Baro Altimeter/1(Altitude) -> Baro Alt (m)/1
  Temperature/1 -> Temp Compensate Baro/1(Temp)

== system SLUGS_Library/Sensor Blocks/Pitot Control End ==
  dyn P [Pa] : Inport
  H_m [m] : Inport  Port=2
  " 0.3 sec tau for high speeds" : Subsystem  mask(Tustin1stOrderLowpassAutoInitialCondition){f=1, T=T}
      mask prompts: f "Lowpass Frequency"; T "Sample Time"
      mask help: Takes a 3db rolloff frequency (in Hz, NOT radians/s) and a sample time. Performs a symbolic Tustin conversion and implements in a discrete filter. The initial output of the filter is set by the first sample.
      mask Help: Enter the desired 3db rolloff frequency in Hz and the sample time. Initial conditions are sampled automatically.
      mask Display: fprintf('%.2f Hz lowpass',f)
  Air Density from Height : Subsystem
  Compute Airspeed : Subsystem
  Protect NaN : Subsystem
  Schedule LPF : Switch  Criteria=u2 > Threshold  Threshold=0.3  OutDataTypeStr=single
  lowpass limit : simulink/Logic and Bit Operations/Compare To Constant  relop=<=  const=5  OutDataTypeStr=uint8  ZeroCross=off
  AirSpeed[m/s] : Outport
  wires:
  Protect NaN/1(Out1) -> Schedule LPF/1, lowpass limit/1, " 0.3 sec tau for high speeds"/1(In1)
  " 0.3 sec tau for high speeds"/1(Out1) -> Schedule LPF/3
  lowpass limit/1 -> Schedule LPF/2
  Compute Airspeed/1(Airspeed m(s)) -> Protect NaN/1(In1)
  Air Density from Height/1(rho (Kg/m^3)) -> Compute Airspeed/2(rho)
  dyn P [Pa]/1 -> Compute Airspeed/1(Dyn P)
  Schedule LPF/1 -> AirSpeed[m/s]/1
  H_m [m]/1 -> Air Density from Height/1(h(m))

== system SLUGS_Library/Sensor Blocks/Pitot Sensor End ==
  Temp : Inport
  DynamicRaw : Inport  Port=2
  Data Type Conversion3 : DataTypeConversion  OutDataTypeStr=double
  Data Type Conversion4 : DataTypeConversion  OutDataTypeStr=single
  Pitot Unit Conversion : Subsystem  mask{bias=pitotOffset, gains=pitotScale}
      mask prompts: bias "Initial Bias"; gains "Initial Gains"
      mask help: Convert Analog readings to units
  Temp Compensate Accel X1 : Subsystem
  "Tustin Lowpass, Auto Initial Condition3" : Subsystem  mask(Tustin1stOrderLowpassAutoInitialCondition){f=pressureSensorCutoff, T=apSampleTime}
      mask prompts: f "Lowpass Frequency"; T "Sample Time"
      mask help: Takes a 3db rolloff frequency (in Hz, NOT radians/s) and a sample time. Performs a symbolic Tustin conversion and implements in a discrete filter. The initial output of the filter is set by the first sample.
      mask Help: Enter the desired 3db rolloff frequency in Hz and the sample time. Initial conditions are sampled automatically.
      mask Display: fprintf('%.2f Hz lowpass',f)
  "[0.001  maxDynPress]" : Saturate  UpperLimit=maxDynPressure  LowerLimit=0.001
  Pitot(Pa) : Outport
  wires:
  Data Type Conversion3/1 -> "Tustin Lowpass, Auto Initial Condition3"/1(In1)
  "Tustin Lowpass, Auto Initial Condition3"/1(Out1) -> Data Type Conversion4/1
  Data Type Conversion4/1 -> Pitot Unit Conversion/1(Raw)
  Pitot Unit Conversion/1(Comp) -> "[0.001  maxDynPress]"/1
  Temp Compensate Accel X1/1(Baro_c) -> Data Type Conversion3/1
  Temp/1 -> Temp Compensate Accel X1/1(Temp)
  "[0.001  maxDynPress]"/1 -> Pitot(Pa)/1
  DynamicRaw/1 -> Temp Compensate Accel X1/2(Dynamic)

== system SLUGS_Library/Singnal Routing & Conditioning/3D Filter ==
  In1 : Inport
  Demux : Demux  Outputs=3
  Filter1 : Subsystem  mask(DiscretizedZeroPole){Zeros=zval, Poles=pval, Gain=kval, AbsTol=auto, SampleTime=TSample, method=tustin, Wc=1}
      mask prompts: Zeros "Zeros (enter in s-main:)"; Poles "Poles (enter in s-domain:)"; Gain "Gain (enter in s-domain:)"; AbsTol "Absolute tolerance:"; SampleTime "Sample time:"; Wc "Critical Frequency (Hz):"
      mask help: Continuous mask uses c2d to transform parameters onto the Discrete Zero-Pole block inside.
      mask init: same as SLUGS_Library/Singnal Routing & Conditioning/Filter
      mask StyleString: edit,edit,edit,edit,edit,popup(zoh|foh|tustin|prewarp|matched),edit
      mask CallbackString: |||||hidecrit|
      mask Display:
      | droots(zeross,poless,gainss)
      | text( 0.5, 1.0, method, 'verticalAlignment','top')
  Filter2 : Subsystem  mask(DiscretizedZeroPole){Zeros=zval, Poles=pval, Gain=kval, AbsTol=auto, SampleTime=TSample, method=tustin, Wc=1}
      mask prompts: Zeros "Zeros (enter in s-main:)"; Poles "Poles (enter in s-domain:)"; Gain "Gain (enter in s-domain:)"; AbsTol "Absolute tolerance:"; SampleTime "Sample time:"; Wc "Critical Frequency (Hz):"
      mask help: Continuous mask uses c2d to transform parameters onto the Discrete Zero-Pole block inside.
      mask init: same as SLUGS_Library/Singnal Routing & Conditioning/Filter
      mask StyleString: edit,edit,edit,edit,edit,popup(zoh|foh|tustin|prewarp|matched),edit
      mask CallbackString: |||||hidecrit|
      mask Display:
      | droots(zeross,poless,gainss)
      | text( 0.5, 1.0, method, 'verticalAlignment','top')
  Filter3 : Subsystem  mask(DiscretizedZeroPole){Zeros=zval, Poles=pval, Gain=kval, AbsTol=auto, SampleTime=TSample, method=tustin, Wc=1}
      mask prompts: Zeros "Zeros (enter in s-main:)"; Poles "Poles (enter in s-domain:)"; Gain "Gain (enter in s-domain:)"; AbsTol "Absolute tolerance:"; SampleTime "Sample time:"; Wc "Critical Frequency (Hz):"
      mask help: Continuous mask uses c2d to transform parameters onto the Discrete Zero-Pole block inside.
      mask init: same as SLUGS_Library/Singnal Routing & Conditioning/Filter
      mask StyleString: edit,edit,edit,edit,edit,popup(zoh|foh|tustin|prewarp|matched),edit
      mask CallbackString: |||||hidecrit|
      mask Display:
      | droots(zeross,poless,gainss)
      | text( 0.5, 1.0, method, 'verticalAlignment','top')
  myMux Fun1 : MATLAB Function  TreatAsAtomicUnit=on
  Out1 : Outport
  wires:
  Demux/1 -> Filter1/1(In1)
  Demux/2 -> Filter2/1(In1)
  Demux/3 -> Filter3/1(In1)
  Filter1/1(Out1) -> myMux Fun1/1(u1)
  Filter2/1(Out1) -> myMux Fun1/2(u2)
  Filter3/1(Out1) -> myMux Fun1/3(u3)
  In1/1 -> Demux/1
  myMux Fun1/1(y) -> Out1/1

== system SLUGS_Library/Singnal Routing & Conditioning/3D LowPass w/Initial Condition ==
  In : Inport
  Demux : Demux  Outputs=3
  Discrete Low Pass : Subsystem  mask{a=a, Yo=yo(1), Ts=T}
      mask prompts: a "Pole location (continuous)"; Yo "Initial condition"; Ts "Sample Time (seconds)"
      mask Display:
      | port_label('input',1,'U')
      | port_label('output',1,'Y')
      | text(0.35,0.85,'Tustin')
      | dpoly([a],[1 a],'s')
  Discrete Low Pass1 : Subsystem  mask{a=a, Yo=yo(2), Ts=T}
      mask prompts: a "Pole location (continuous)"; Yo "Initial condition"; Ts "Sample Time (seconds)"
      mask Display:
      | port_label('input',1,'U')
      | port_label('output',1,'Y')
      | text(0.35,0.85,'Tustin')
      | dpoly([a],[1 a],'s')
  Discrete Low Pass2 : Subsystem  mask{a=a, Yo=yo(3), Ts=T}
      mask prompts: a "Pole location (continuous)"; Yo "Initial condition"; Ts "Sample Time (seconds)"
      mask Display:
      | port_label('input',1,'U')
      | port_label('output',1,'Y')
      | text(0.35,0.85,'Tustin')
      | dpoly([a],[1 a],'s')
  myMux Fun1 : MATLAB Function  TreatAsAtomicUnit=on
  Out1 : Outport
  wires:
  Discrete Low Pass2/1(Y) -> myMux Fun1/3(u3)
  Discrete Low Pass1/1(Y) -> myMux Fun1/2(u2)
  Discrete Low Pass/1(Y) -> myMux Fun1/1(u1)
  myMux Fun1/1(y) -> Out1/1
  Demux/1 -> Discrete Low Pass/1(U)
  Demux/2 -> Discrete Low Pass1/1(U)
  Demux/3 -> Discrete Low Pass2/1(U)
  In/1 -> Demux/1

== system SLUGS_Library/Singnal Routing & Conditioning/Discrete Low Pass w/initial condition ==
  U : Inport
  Gain : Gain  Gain=(2-a*Ts)  SampleTime=Ts
  Gain1 : Gain  Gain=1/(2+a*Ts)  SampleTime=Ts
  Gain2 : Gain  Gain=a*Ts  SampleTime=Ts
  Sum : Sum  Inputs=++|
  Sum1 : Sum  Inputs=|++
  Unit Delay : UnitDelay  X0=Yo  SampleTime=Ts
  Unit Delay1 : UnitDelay  X0=Yo  SampleTime=Ts
  Y : Outport
  wires:
  Gain/1 -> Sum1/2
  Sum1/1 -> Gain1/1
  Gain2/1 -> Sum1/1
  Gain1/1 -> Y/1, Unit Delay/1  "Y_k"
  Sum/1 -> Gain2/1
  Unit Delay1/1 -> Sum/2  "U_k-1"
  U/1 -> Sum/1, Unit Delay1/1  "U_k"
  Unit Delay/1 -> Gain/1  "Y_k-1"

== system SLUGS_Library/Singnal Routing & Conditioning/Ellipse Correction ==
  note: x = (x - param.xo) ./ param.a;
  note: y = (((y - param.yo) ./ param.b) - x.*sin(deg2rad(param.phi))) ./ cos(deg2rad(param.phi));
  note: z = (((z - param.zo) ./ param.c) - x.*sin(deg2rad(param.row)).*cos(deg2rad(param.lambda)) - y.*sin(deg2rad(param.lambda))) ./ (cos(deg2rad(param.row))*cos(deg2rad(param.lambda)));
  Raw : Inport
  Constant : Constant  Value=param.xo
  Constant1 : Constant  Value=param.yo
  Constant2 : Constant  Value=param.phi_rad  OutDataTypeStr=single
  Constant3 : Constant  Value=param.zo
  Constant4 : Constant  Value=param.rho_rad  OutDataTypeStr=single
  Constant5 : Constant  Value=param.lambda_rad  VectorParams1D=off  OutDataTypeStr=single
  Demux : Demux  Outputs=3
  Gain : Gain  Gain=param.one_over_a
  Gain1 : Gain  Gain=param.one_over_b
  Gain2 : Gain  Gain=param.one_over_c
  Product{,1..3} (4 alike) : Product  RndMeth=Zero
  Product4 : Product  Inputs=*//  RndMeth=Zero
  Subsystem1 : Subsystem  AncestorBlock=SLUGS_Library/Subsystem5
  Subsystem5 : Subsystem  AncestorBlock=SLUGS_Library/Subsystem5
  Subsystem8 : Subsystem  AncestorBlock=SLUGS_Library/Subsystem8
  Sum : Sum  Inputs=-+|
  Sum1 : Sum  Inputs=|+-
  Sum2 : Sum  Inputs=-+|
  Sum3 : Sum  Inputs=|+-
  Sum4 : Sum  Inputs=-+-
  myMux Fun3 : MATLAB Function  AncestorBlock=SLUGS_Library/Singnal Routing & Conditioning/myMux Fun3  TreatAsAtomicUnit=on
  Corr : Outport
  wires:
  Raw/1 -> Demux/1
  Demux/1 -> Sum/2
  Constant/1 -> Sum/1
  Sum/1 -> Gain/1
  Gain/1 -> [X], Product/1, myMux Fun3/1(u1)
  Sum1/1 -> Gain1/1
  myMux Fun3/1(y) -> Corr/1
  Constant1/1 -> Sum1/2
  Demux/2 -> Sum1/1
  Constant2/1 -> Subsystem8/1(x)
  Subsystem8/1(tan(x)) -> [Tan_Phi]
  [Tan_Phi] -> Product/2
  Gain1/1 -> Sum2/2
  Product/1 -> Sum2/1
  Sum2/1 -> [Y], myMux Fun3/2(u2)
  Sum3/1 -> Gain2/1
  Constant3/1 -> Sum3/2
  Gain2/1 -> Sum4/2
  Demux/3 -> Sum3/1
  Constant4/1 -> Subsystem5/1(u)
  Constant5/1 -> Subsystem1/1(u)
  Subsystem5/1(sin(u)) -> Product1/1
  Subsystem1/2(cos(u)) -> Product1/2, Product4/3
  Product1/1 -> [Sin_rho_Cos_lam]
  [X] -> Product2/1
  [Sin_rho_Cos_lam] -> Product2/2
  Product2/1 -> Sum4/1
  [Y] -> Product3/1
  [slam_crhoclam] -> Product3/2
  Product3/1 -> Sum4/3
  Subsystem1/1(sin(u)) -> Product4/1
  Subsystem5/2(cos(u)) -> Product4/2
  Product4/1 -> [slam_crhoclam]
  Sum4/1 -> myMux Fun3/3(u3)

== system SLUGS_Library/Singnal Routing & Conditioning/Filter ==
  In1 : Inport
  Discrete Zero-Pole : DiscreteZeroPole  Zeros=zerosd  Poles=polesd  Gain=gaind  SampleTime=SampleTime
  Out1 : Outport
  wires:
  Discrete Zero-Pole/1 -> Out1/1
  In1/1 -> Discrete Zero-Pole/1
